simulink model "DigitalDesign"  (R2023a)
settings: Solver=VariableStepAuto  StartTime=0.0  StopTime=inf  RelTol=1e-3
model workspace (MAT data in the model file):
  Period = Simulink.Parameter
  Period.Value = 2
  Period.DataType = 'auto'
  Period.Complexity = 'real'
  Period.Dimensions = [1 1]
settings Model: Creator=User  LastModifiedBy=User

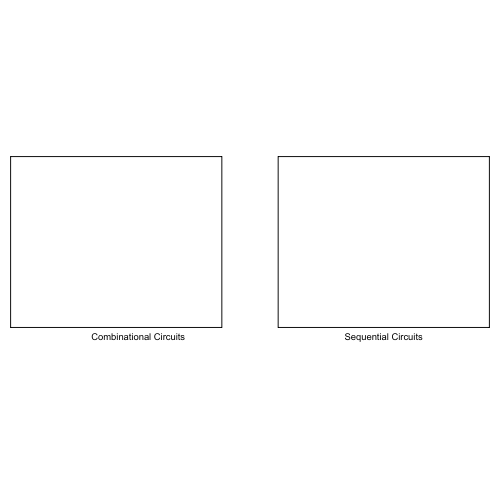
[thumbnail: Simulink's stored preview of the top-level diagram]
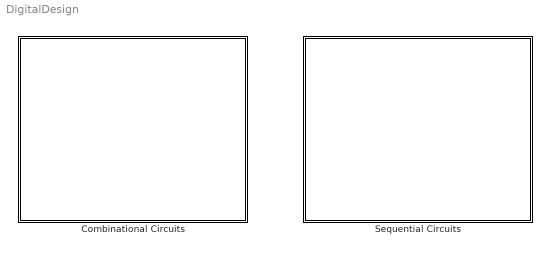
== system DigitalDesign ==
  "                 Combinational Circuits" : Subsystem
  Sequential Circuits : Subsystem

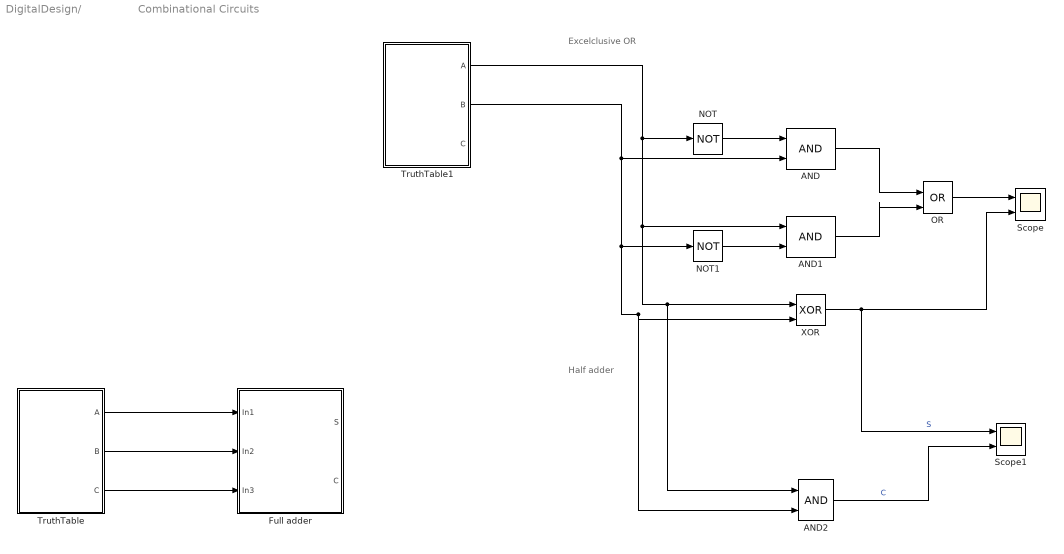
== system DigitalDesign/                 Combinational Circuits ==
  note: Excelclusive OR
  note: Half adder
  AND : Logic  IconShape=distinctive  AllPortsSameDT=off  OutDataTypeStr=boolean
  AND1 : Logic  IconShape=distinctive  AllPortsSameDT=off  OutDataTypeStr=boolean
  AND2 : Logic  IconShape=distinctive  AllPortsSameDT=off  OutDataTypeStr=boolean
  Full adder : Subsystem
  NOT : Logic  Operator=NOT  IconShape=distinctive  AllPortsSameDT=off  OutDataTypeStr=boolean
  NOT1 : Logic  Operator=NOT  IconShape=distinctive  AllPortsSameDT=off  OutDataTypeStr=boolean
  OR : Logic  Operator=OR  IconShape=distinctive  AllPortsSameDT=off  OutDataTypeStr=boolean
  Scope : Scope  NumInputPorts=2
  Scope1 : Scope  NumInputPorts=2
  TruthTable : Subsystem
  TruthTable1 : Subsystem
  XOR : Logic  Operator=XOR  IconShape=distinctive  AllPortsSameDT=off  OutDataTypeStr=boolean
  wires:
  AND2/1 -> Scope1/2  "C"
  TruthTable/3(C) -> Full adder/3(In3)
  AND/1 -> OR/1
  TruthTable/1(A) -> Full adder/1(In1)
  AND1/1 -> OR/2
  TruthTable1/2(B) -> AND2/2, XOR/2, NOT1/1, AND/2
  TruthTable1/1(A) -> AND2/1, XOR/1, AND1/1, NOT/1
  NOT1/1 -> AND1/2
  XOR/1 -> Scope1/1, Scope/2  "S"
  OR/1 -> Scope/1
  TruthTable/2(B) -> Full adder/2(In2)
  NOT/1 -> AND/1

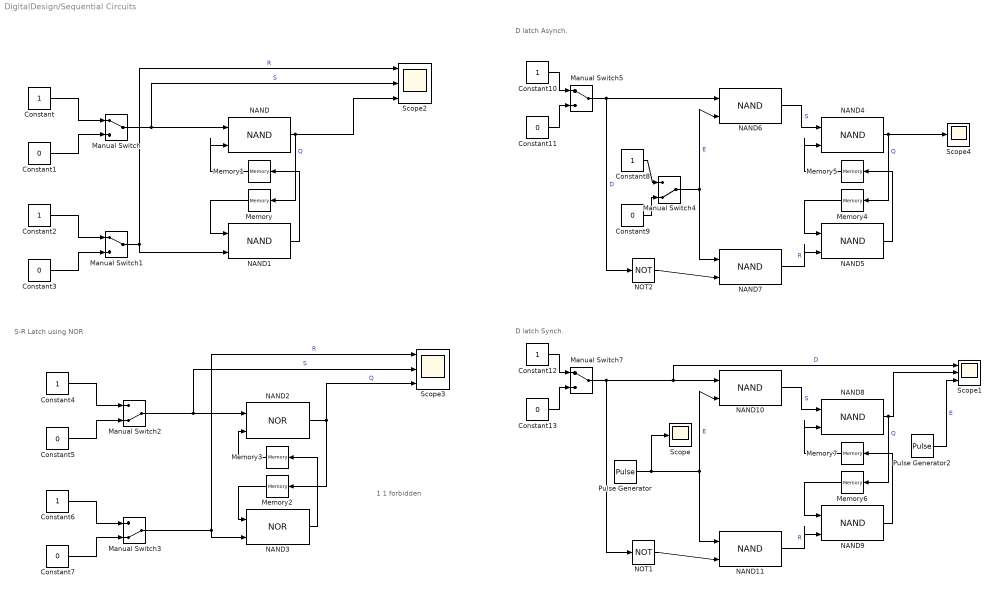
== system DigitalDesign/Sequential Circuits ==
  note: D latch Asynch.
  note: S-R Latch using NOR
  note: 1 1 forbidden
  note: D latch Synch.
  Constant{,2,4,6,8,10,12} (7 alike) : Constant
  Constant{1,3,5,7,9,11,13} (7 alike) : Constant  Value=0
  Manual Switch{,1,5,7} (4 alike) : ManualSwitch
  Manual Switch2 : ManualSwitch  CurrentSetting=0
  Manual Switch3 : ManualSwitch  CurrentSetting=0
  Manual Switch4 : ManualSwitch  CurrentSetting=0
  Memory{,1..7} (8 alike) : Memory
  NAND{,1,4..11} (10 alike) : Logic  Operator=NAND  IconShape=distinctive  AllPortsSameDT=off  OutDataTypeStr=boolean
  NAND2 : Logic  Operator=NOR  IconShape=distinctive  AllPortsSameDT=off  OutDataTypeStr=boolean
  NAND3 : Logic  Operator=NOR  IconShape=distinctive  AllPortsSameDT=off  OutDataTypeStr=boolean
  NOT1 : Logic  Operator=NOT  IconShape=distinctive  AllPortsSameDT=off  OutDataTypeStr=boolean
  NOT2 : Logic  Operator=NOT  IconShape=distinctive  AllPortsSameDT=off  OutDataTypeStr=boolean
  Pulse Generator : DiscretePulseGenerator  PulseType=Time based  PulseWidth=5
  Pulse Generator2 : DiscretePulseGenerator  PulseType=Time based  PulseWidth=5
  Scope : Scope
  Scope1 : Scope  NumInputPorts=3
  Scope2 : Scope  NumInputPorts=3
  Scope3 : Scope  NumInputPorts=3
  Scope4 : Scope
  wires:
  NOT2/1 -> NAND7/2
  Manual Switch5/1 -> NOT2/1, NAND6/1  "D"
  NAND4/1 -> Scope4/1, Memory4/1  "Q"
  Memory4/1 -> NAND5/1
  Memory5/1 -> NAND4/2
  NAND7/1 -> NAND5/2  "R"
  Constant11/1 -> Manual Switch5/2
  NAND2/1 -> Scope3/3, Memory2/1  "Q"
  Constant10/1 -> Manual Switch5/1
  Manual Switch3/1 -> NAND3/2, Scope3/1  "R"
  Constant7/1 -> Manual Switch3/2
  Constant6/1 -> Manual Switch3/1
  NAND3/1 -> Memory3/1
  Memory2/1 -> NAND3/1
  Constant3/1 -> Manual Switch1/2
  Manual Switch2/1 -> NAND2/1, Scope3/2  "S"
  Constant4/1 -> Manual Switch2/1
  Constant1/1 -> Manual Switch/2
  NAND5/1 -> Memory5/1
  Memory3/1 -> NAND2/2
  Memory/1 -> NAND1/1
  Constant8/1 -> Manual Switch4/1
  Constant/1 -> Manual Switch/1
  Constant2/1 -> Manual Switch1/1
  Manual Switch1/1 -> Scope2/1, NAND1/2  "R"
  NAND1/1 -> Memory1/1
  NAND6/1 -> NAND4/1  "S"
  Constant5/1 -> Manual Switch2/2
  Memory1/1 -> NAND/2
  Constant9/1 -> Manual Switch4/2
  NAND/1 -> Memory/1, Scope2/3  "Q"
  Manual Switch4/1 -> NAND6/2, NAND7/1  "E"
  Manual Switch/1 -> Scope2/2, NAND/1  "S"
  Pulse Generator/1 -> Scope/1, NAND11/1, NAND10/2  "E"
  NAND10/1 -> NAND8/1  "S"
  NAND9/1 -> Memory7/1
  Constant12/1 -> Manual Switch7/1
  Constant13/1 -> Manual Switch7/2
  NAND11/1 -> NAND9/2  "R"
  Memory7/1 -> NAND8/2
  Memory6/1 -> NAND9/1
  NAND8/1 -> Memory6/1, Scope1/2  "Q"
  Manual Switch7/1 -> Scope1/1, NAND10/1, NOT1/1  "D"
  NOT1/1 -> NAND11/2
  Pulse Generator2/1 -> Scope1/3  "E"

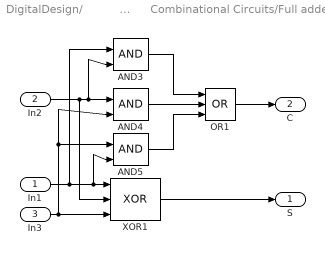
== system DigitalDesign/                 Combinational Circuits/Full adder ==
  In1 : Inport
  In2 : Inport  Port=2
  In3 : Inport  Port=3
  AND3 : Logic  IconShape=distinctive  AllPortsSameDT=off  OutDataTypeStr=boolean
  AND4 : Logic  IconShape=distinctive  AllPortsSameDT=off  OutDataTypeStr=boolean
  AND5 : Logic  IconShape=distinctive  AllPortsSameDT=off  OutDataTypeStr=boolean
  OR1 : Logic  Operator=OR  Inputs=3  IconShape=distinctive  AllPortsSameDT=off  OutDataTypeStr=boolean
  XOR1 : Logic  Operator=XOR  Inputs=3  IconShape=distinctive  AllPortsSameDT=off  OutDataTypeStr=boolean
  S : Outport
  C : Outport  Port=2
  wires:
  OR1/1 -> C/1
  AND5/1 -> OR1/3
  In1/1 -> AND5/2, XOR1/1, AND3/1
  In2/1 -> AND3/2, AND4/1, XOR1/2
  In3/1 -> AND4/2, AND5/1, XOR1/3
  AND3/1 -> OR1/1
  AND4/1 -> OR1/2
  XOR1/1 -> S/1

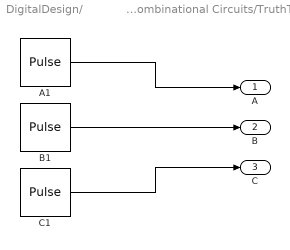
== system DigitalDesign/                 Combinational Circuits/TruthTable ==
  A1 : DiscretePulseGenerator  PulseType=Time based  Period=Period*4  PulseWidth=50  PhaseDelay=.5*Period*4
  B1 : DiscretePulseGenerator  PulseType=Time based  Period=Period*2  PulseWidth=50  PhaseDelay=.5*Period*2
  C1 : DiscretePulseGenerator  PulseType=Time based  Period=Period  PulseWidth=50  PhaseDelay=.5*Period
  A : Outport
  B : Outport  Port=2
  C : Outport  Port=3
  wires:
  B1/1 -> B/1
  A1/1 -> A/1
  C1/1 -> C/1

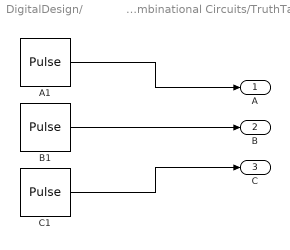
== system DigitalDesign/                 Combinational Circuits/TruthTable1 ==
  A1 : DiscretePulseGenerator  PulseType=Time based  Period=Period*4  PulseWidth=50  PhaseDelay=.5*Period*4
  B1 : DiscretePulseGenerator  PulseType=Time based  Period=Period*2  PulseWidth=50  PhaseDelay=.5*Period*2
  C1 : DiscretePulseGenerator  PulseType=Time based  Period=Period  PulseWidth=50  PhaseDelay=.5*Period
  A : Outport
  B : Outport  Port=2
  C : Outport  Port=3
  wires:
  C1/1 -> C/1
  A1/1 -> A/1
  B1/1 -> B/1
